simulink model "REI_Ubicacion"  (R2021a)
settings: Solver=VariableStepAuto  StartTime=0.0  StopTime=20  RelTol=1e-3
values from neighbouring files (symbols this model uses):
  Ac = [0, 1; -tf3.denominator{1}(3), -tf3.denominator{1}(2)]    [modelo.m]
  Bc = [0; tf3.numerator{1}(3)]    [modelo.m]
  Cc = [1, 0]    [modelo.m]
  K12 = Ks(1:2)    [modelo.m]
  K3 = -Ks(3)    [modelo.m]
undefined symbols (not defined in the file or in its folder): sigbuilder_block
settings Model: Creator=dherr  LastModifiedBy=dherr
settings DataIOCC: ReturnWorkspaceOutputs=off

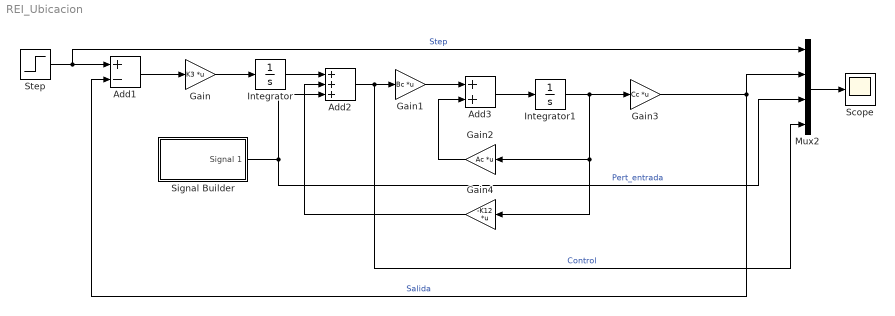
== system REI_Ubicacion ==
  Add1 : Sum  Inputs=+-
  Add2 : Sum  Inputs=+++
  Add3 : Sum
  Gain : Gain  Gain=K3  Multiplication=Matrix(K*u)
  Gain1 : Gain  Gain=Bc  Multiplication=Matrix(K*u)
  Gain2 : Gain  Gain=Ac  Multiplication=Matrix(K*u)
  Gain3 : Gain  Gain=Cc  Multiplication=Matrix(K*u)
  Gain4 : Gain  Gain=-K12  Multiplication=Matrix(K*u)
  Integrator : Integrator
  Integrator1 : Integrator
  Mux2 : Mux
  Scope : Scope
  Signal Builder : Subsystem  Tag=STV Subsys  LoadFcn=sigbuilder_block('load');  StartFcn=sigbuilder_block('start');  StopFcn=sigbuilder_block('stop');  ClipboardFcn=sigbuilder_block('clipboard');  mask(Sigbuilder block){tuvar=[0:10]}
      mask help: Simulink:masks:SigbuilderBlock_MD
      mask init:
      | if ~strcmp(get_param(bdroot(gcbh),'SimulationStatus'),'stopped') tuvar = sigbuilder_block('maskInit'); end
      settings: CopyFcn=sigbuilder_block('copy');  DeleteFcn=sigbuilder_block('delete');  ModelCloseFcn=sigbuilder_block('modelClose');  PreSaveFcn=sigbuilder_block('preSave');  PauseFcn=sigbuilder_block('pause');  ContinueFcn=sigbuilder_block('continue');  NameChangeFcn=sigbuilder_block('namechange');  OpenFcn=sigbuilder_block('open',[448.2 138.6 550.8 400.2 ]);  CloseFcn=sigbuilder_block('close');
      mask Display: plot(0, 0, 100, 100,[2, 2, 32, 32, 2], [68, 8, 8, 68, 68],[32, 2], [38, 38], [32, 19, 2],[53, 60, 44], [32, 17, 17, 2],[16, 16, 31, 31]);txt = getActiveGroup(gcbh);text(2, 100, txt,'verticalAlignment', 'top');
  Step : Step  After=0.6  SampleTime=0
  wires:
  Mux2/1 -> Scope/1
  Add3/1 -> Integrator1/1
  Step/1 -> Mux2/1, Add1/1  "Step"
  Gain2/1 -> Add3/2
  Add2/1 -> Mux2/4, Gain1/1  "Control"
  Integrator1/1 -> Gain3/1, Gain4/1, Gain2/1
  Gain4/1 -> Add2/2
  Gain1/1 -> Add3/1
  Add1/1 -> Gain/1
  Gain/1 -> Integrator/1
  Integrator/1 -> Add2/1
  Signal Builder/1(Signal 1) -> Add2/3, Mux2/3  "Pert_entrada"
  Gain3/1 -> Add1/2, Mux2/2  "Salida"

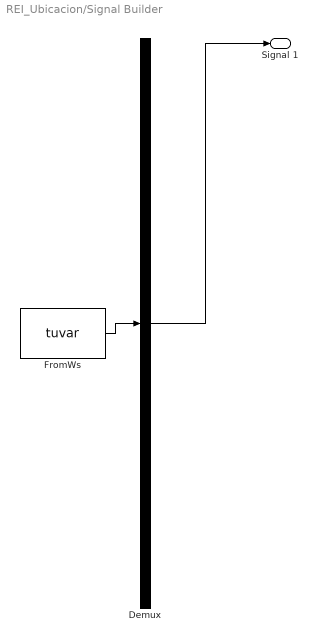
== system REI_Ubicacion/Signal Builder ==
  Demux : Demux  Tag=STV Demux  Outputs=1
      settings: DisplayOption=none
  FromWs : FromWorkspace  Tag=STV FromWs  VariableName=tuvar
      SigBuilderData=|
      | common.afterFinalStr = 'Extrapolate'
      | common.sampleTime = 0
      | dataSet.timeRange = [0 20]
      | dataSet.name = 'Group 1'
      | sbobj.Groups.Name = 'Group 1'
      | sbobj.Groups.Signals.Name = 'Signal 1'
      | sbobj.Groups.Signals.XData = [0 9 9 15 15 20]
      | sbobj.Groups.Signals.YData = [0 0 0.1 0.1 0 0]
      | sbobj.Groups.TimeRange = [0 20]
  Signal 1 : Outport  Tag=STV Outport
  wires:
  Demux/1 -> Signal 1/1
  FromWs/1 -> Demux/1
